simulink model "water_4hopper"  (Simulink 8.0)
settings: Solver=ode23  StartTime=0.0  StopTime=30  RelTol=1e-3
values from neighbouring files (symbols this model uses):
  Ac = [sum(Ay), sum(Ath), sum(Aph) ... (first row only)    [simpleSys.m]
  alpha = 1/16    (= 0.0625)    [simpleSys.m]
  C_d = 0.703    [simpleSys.m]
  density = 1000    [simpleSys.m]
  Filter_Coef = 1000    [simpleSys.m]
  g = 9.81    [simpleSys.m]
  Gc = [sum(G) - mass*g ; Lx'*G ; Lz'*G]    [simpleSys.m]
  mass = 0.15    [simpleSys.m]
  nullProj = eye(8) - pinvBc*Bc    [simpleSys.m]
  phi = 0 * pi/180    (= 0)    [simpleSys.m]
  pinvBc = pinv(Bc)    [simpleSys.m]
  S1 = pi*r1^2*area    (= 0.000684741534776)    [simpleSys.m]
  S2 = pi*r2^2*area    (= 4.27963459235e-05)    [simpleSys.m]
  theta = 0 * pi/180    (= 0)    [simpleSys.m]
  w = 60    [simpleSys.m]
  y = 0.020    (= 0.02)    [simpleSys.m]
undefined symbols (not defined in the file or in its folder): dTorqueAmp, dTorqueFreq, dTorquePhase, frame_inertia, freq, Kdf, leg_length, Mc, omega_0, tau, waveAmp, waveFreq
undefined symbols (not defined in the file): amp, cw_FL_HL, cw_FR_FL, cw_FR_HR, cw_HR_HL, FL_HL_lag, FR_FL_lag, FR_HR_lag, HR_HL_lag, K_d, K_i, K_p, wavePhase
libraries: mblibv1 x31, dspstat3 x6
(part 1 of 2)
settings Model: Creator=Metti  LastModifiedBy=nitisht  SimulationMode=accelerator
settings SolverCC: ZeroCrossControl=DisableAll
settings DataIOCC: SignalLoggingSaveFormat=ModelDataLogs
settings DebuggingCC: FcnCallInpInsideContextMsg=EnableAllAsWarning
settings SimMechanicsCC: VisSampleTime=0.05  AutoFitVis=GROWTOFIT  LastVizWinPosition=[1 41 1600 759]  CamPosition=[-6.20117;3.01965;9.86212;]  CamTarget=[-0.265896;0.0450483;0.16365;]  CamUpVector=[0.0887544;0.966202;-0.242026;]  CamHeight=0.984746  VisBackgroundColor=[0.9;0.9;0.95;]  DefaultBodyColor=[1;0;0;]
settings ConfigurationSet: Description=SimMechanics 2G

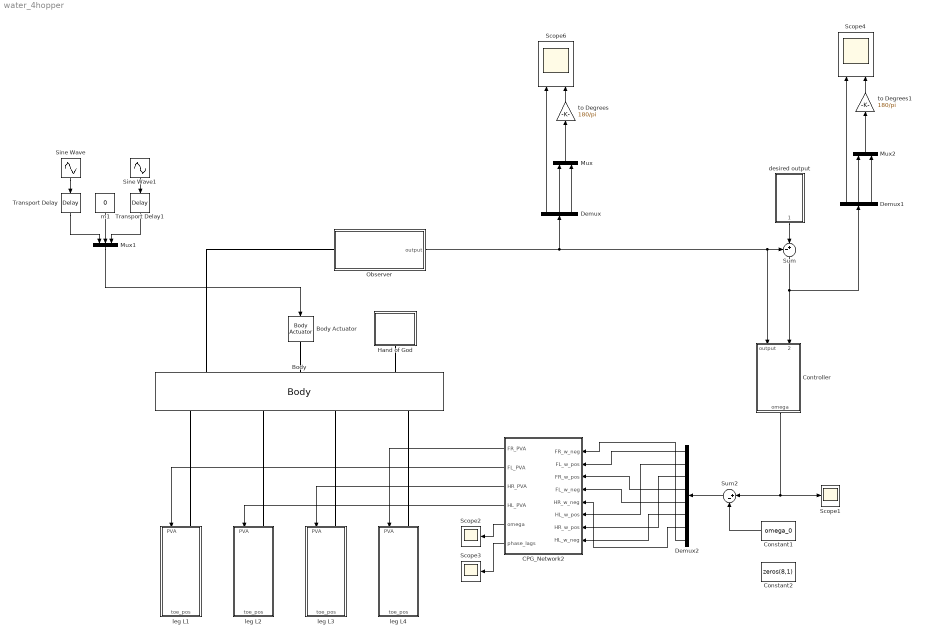
== system water_4hopper ==
  Body : mblibv1/Bodies/Body  LConnTagsString=CG|CS10|CS1  RConnTagsString=CS2|CS3|CS4|CS5  UpdateFromCAD=off  DialogClass=MechanicalBodyBlock  Mass=mass  MassUnits=kg  InertiaUnits=kg*m^2  Inertia=frame_inertia  Shape=Cylinder  ShapeDims=[1 1]  ShapeUnits=m  ShapeUse=false  Density=1  DensityUnits=kg/m^3  DensityUse=false  GraphicsMode=MACHINE_DEFAULT  BodyColorSelMode=MACHINE_DEFAULT  BodyColor=[1 0 0]  AttachedToCS=CG  CG=Left$CG$CG_pos$CS1$CS1$m$[0 0 0]$Euler X-Y-Z$deg$WORLD$true$none  WorkingFrames=Left$CS10$CG_pos$CS1$CS1$m$[0 0 0]$Euler X-Y-Z$deg$WORLD$true$none#Left$CS1$[0 0 0]$Adjoining$Adjoining$m$[0 0 0]$Euler X-Y-Z$deg$WORLD$true$none#Right$CS2$TR_FL$CS1$CS1$m$[0 0 0]$Euler X-Y-Z$deg$WORLD$true$none#Right$CS3$TR_HL$CS1$CS1$m$[0 0 0]$Euler X-Y-Z$deg$WORLD$true$none#Right$CS4$TR_HR$CS1$CS1$m$[0 0 0]$Euler X-Y-Z$deg$WORLD$true$none#Right$CS5$TR_FR$CS1$CS1$m$[0 0 0]$Euler X-Y-Z$deg$WORLD$true$none  CGPos=CG_pos  CGRot=[0 0 0]  CS0Pos=[]  CS0Rot=[]  CS1Pos=[0 0 0]  CS1Rot=[0 0 0]  CS2Pos=TR_FL  CS2Rot=[0 0 0]  CS3Pos=TR_HL  CS3Rot=[0 0 0]  CS4Pos=TR_HR  CS4Rot=[0 0 0]  CS5Pos=TR_FR  CS5Rot=[0 0 0]  CS6Pos=[]  CS6Rot=[]  CS7Pos=[]  CS7Rot=[]  CS8Pos=[]  CS8Rot=[]  CS9Pos=[]  CS9Rot=[]  CS10Pos=CG_pos  CS10Rot=[0 0 0]  CS11Pos=[]  CS11Rot=[]  CS12Pos=[]  CS12Rot=[]  CS13Pos=[]  CS13Rot=[]  CS14Pos=[]  CS14Rot=[]  CS15Pos=[]  CS15Rot=[]  CS16Pos=[]  CS16Rot=[]  CS17Pos=[]  CS17Rot=[]  CS18Pos=[]  CS18Rot=[]  CS19Pos=[]  CS19Rot=[]  CS20Pos=[]  CS20Rot=[]
  Body Actuator : mblibv1/Sensors &  Actuators/Body Actuator  UpdateFromCAD=off  PhysicalDomain=Mechanical  PortType=blob  ActuationStyle=Force  AngleUnits=deg  ArcVelocityUnits=deg/s  ArcAccelerationUnits=deg/s^2  CoordPositionUnits=m  VelocityUnits=m/s  AccelerationUnits=m/s^2  ForceUnits=N  TorqueUnits=N*m  ActiveIO=on  Width=3  DialogClass=MechanicalActuatorBlock  ReferenceFrame=Absolute (World)  Angle=off  CoordPosition=on  Force=off  Torque=on
  CPG_Network2 : Subsystem
  Constant1 : Constant  Value=omega_0
  Constant2 : Constant  Value=zeros(8,1)
  Controller : Subsystem
  Demux : Demux  Outputs=3
  Demux1 : Demux  Outputs=3
  Demux2 : Demux  Outputs=8
  Hand of God : Subsystem
  Mux : Mux  Inputs=2
  Mux1 : Mux  Inputs=3
  Mux2 : Mux  Inputs=2
  Observer : Subsystem
  Scope1 : Scope
      settings: TimeRange=30  YMin=25  YMax=95  SaveName=command_omega
  Scope2 : Scope
      settings: ShowLegends=on  TimeRange=30  YMin=-10  YMax=120  SaveName=CPG_omega
  Scope3 : Scope
      settings: ShowLegends=on  TimeRange=30  YMin=0  YMax=6.5  SaveName=CPG_phase_lags
  Scope4 : Scope  NumInputPorts=2
      settings: TimeRange=30  YMin=0.0125~-0.0225  YMax=0.0275~0.02  SaveName=ball_position1
  Scope6 : Scope  NumInputPorts=2
      settings: TimeRange=30  YMin=0.0125~-0.0225  YMax=0.0275~0.02  SaveName=ball_position
  Sine Wave : Sin  Amplitude=dTorqueAmp  Frequency=dTorqueFreq  Phase=dTorquePhase(1)  SampleTime=0
  Sine Wave1 : Sin  Amplitude=dTorqueAmp  Frequency=dTorqueFreq  Phase=dTorquePhase(2)  SampleTime=0
  Sum : Sum  Inputs=-+|
  Sum2 : Sum  Inputs=|+-
  Transport Delay : TransportDelay  DelayTime=5
  Transport Delay1 : TransportDelay  DelayTime=5
  desired output : Subsystem
  leg L1 : Subsystem  mask{wphase=wavePhase(1)}
      mask prompts: wphase "wave phase"
  leg L2 : Subsystem  mask{wphase=wavePhase(2)}
      mask prompts: wphase "wave phase"
  leg L3 : Subsystem  mask{wphase=wavePhase(3)}
      mask prompts: wphase "wave phase"
  leg L4 : Subsystem  mask{wphase=wavePhase(4)}
      mask prompts: wphase "wave phase"
  m1 : Constant  Value=0
  to Degrees : Gain  Gain=180/pi
  to Degrees1 : Gain  Gain=180/pi
  wires:
  Demux2/1 -> CPG_Network2/2(FL_w_pos)
  Demux2/5 -> CPG_Network2/4(FL_w_neg)
  Demux2/2 -> CPG_Network2/6(HL_w_pos)
  Demux2/6 -> CPG_Network2/8(HL_w_neg)
  Demux2/3 -> CPG_Network2/7(HR_w_pos)
  Demux2/7 -> CPG_Network2/5(HR_w_neg)
  Demux2/4 -> CPG_Network2/3(FR_w_pos)
  Demux2/8 -> CPG_Network2/1(FR_w_neg)
  CPG_Network2/5(omega) -> Scope2/1
  Sine Wave/1 -> Transport Delay/1
  Mux1/1 -> Body Actuator/1
  Transport Delay/1 -> Mux1/1
  Transport Delay1/1 -> Mux1/3
  m1/1 -> Mux1/2
  Sine Wave1/1 -> Transport Delay1/1
  CPG_Network2/6("phase_lags ") -> Scope3/1
  desired output/1(desired output) -> Sum/2
  Controller/1(omega) -> Scope1/1, Sum2/1
  CPG_Network2/2(FL_PVA) -> leg L1/1(PVA)
  CPG_Network2/4(HL_PVA) -> leg L2/1(PVA)
  CPG_Network2/3(HR_PVA) -> leg L3/1(PVA)
  CPG_Network2/1(FR_PVA) -> leg L4/1(PVA)
  Constant1/1 -> Sum2/2
  Observer/1(output) -> Sum/1, Controller/1(output), Demux/1
  Demux/2 -> Mux/1
  Demux/3 -> Mux/2
  Mux/1 -> to Degrees/1
  to Degrees/1 -> Scope6/2
  Demux/1 -> Scope6/1
  Sum2/1 -> Demux2/1
  Sum/1 -> Demux1/1, Controller/2(output error)
  Demux1/2 -> Mux2/1
  Demux1/3 -> Mux2/2
  Mux2/1 -> to Degrees1/1
  to Degrees1/1 -> Scope4/2
  Demux1/1 -> Scope4/1
  connections:
  Hand of God/RConn1 -- Body/LConn3
  leg L4/LConn1 -- Body/RConn4
  leg L3/LConn1 -- Body/RConn3
  leg L2/LConn1 -- Body/RConn2
  leg L1/LConn1 -- Body/RConn1
  Body Actuator/RConn1 -- Body/LConn2
  Observer/LConn1 -- Body/LConn1

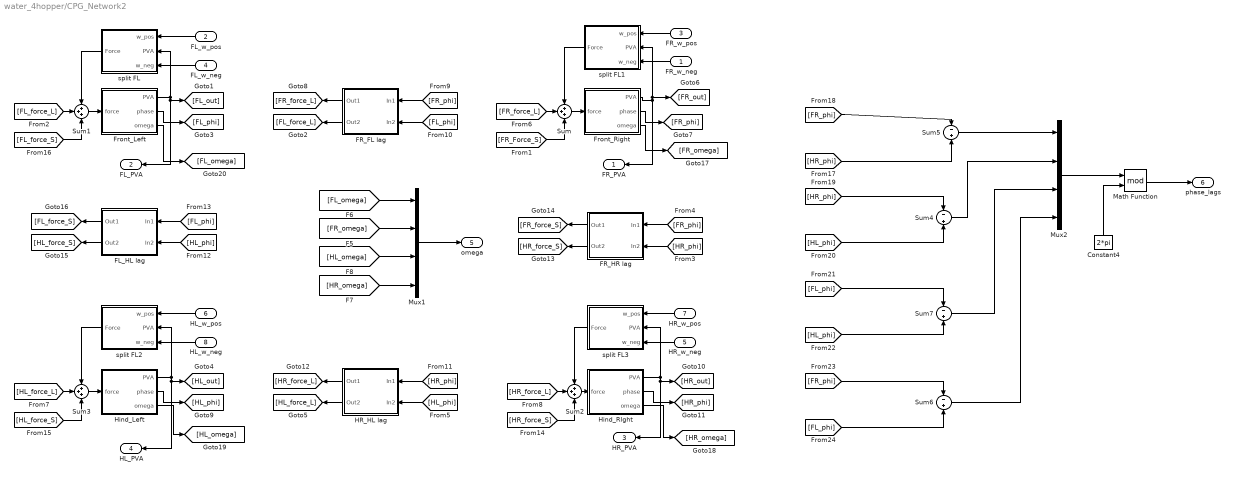
== system water_4hopper/CPG_Network2 ==
  FR_w_neg : Inport
  FL_w_pos : Inport  Port=2
  FR_w_pos : Inport  Port=3
  FL_w_neg : Inport  Port=4
  HR_w_neg : Inport  Port=5
  HL_w_pos : Inport  Port=6
  HR_w_pos : Inport  Port=7
  HL_w_neg : Inport  Port=8
  Constant4 : Constant  Value=2*pi
  FL_HL lag : Subsystem  mask{d_phase=FL_HL_lag, coupling_weight=cw_FL_HL}
      mask prompts: d_phase "Phase Lag"; coupling_weight "Coupling Weight"
  FR_FL lag : Subsystem  mask{d_phase=FR_FL_lag, coupling_weight=cw_FR_FL}
      mask prompts: d_phase "Phase Lag"; coupling_weight "Coupling Weight"
  FR_HR lag : Subsystem  mask{d_phase=FR_HR_lag, coupling_weight=cw_FR_HR}
      mask prompts: d_phase "Phase Lag"; coupling_weight "Coupling Weight"
  Front_Left : Subsystem  mask{Amp=amp, Offset=0, init_phi=pi}
      mask prompts: Amp "Amplitude"; init_phi "Initial Phase"
  Front_Right : Subsystem  mask{Amp=amp, Offset=0, init_phi=0}
      mask prompts: Amp "Amplitude"; init_phi "Initial Phase"
  HR_HL lag : Subsystem  mask{d_phase=HR_HL_lag, coupling_weight=cw_HR_HL}
      mask prompts: d_phase "Phase Lag"; coupling_weight "Coupling Weight"
  Hind_Left : Subsystem  mask{Amp=amp, Offset=0, init_phi=0}
      mask prompts: Amp "Amplitude"; init_phi "Initial Phase"
  Hind_RIght : Subsystem  mask{Amp=amp, Offset=0, init_phi=pi}
      mask prompts: Amp "Amplitude"; init_phi "Initial Phase"
  Math Function : Math  Operator=mod  SaturateOnIntegerOverflow=on
  Mux1 : Mux
  Mux2 : Mux
  Sum{,1..3} (4 alike) : Sum  Inputs=+++
  Sum{4..7} (4 alike) : Sum  Inputs=-|+
  split FL : Subsystem
  split FL1 : Subsystem
  split FL2 : Subsystem
  split FL3 : Subsystem
  FR_PVA : Outport
  FL_PVA : Outport  Port=2
  HR_PVA : Outport  Port=3
  HL_PVA : Outport  Port=4
  omega : Outport  Port=5
  "phase_lags " : Outport  Port=6
  wires:
  Front_Left/2(phase) -> [FL_phi]
  Front_Right/2(phase) -> [FR_phi]
  [FL_phi] -> FR_FL lag/2(In2)
  [FR_phi] -> FR_FL lag/1(In1)
  FR_FL lag/1(Out1) -> [FR_force_L]
  FR_FL lag/2(Out2) -> [FL_force_L]
  Front_Right/1(PVA) -> split FL1/2(PVA), [FR_out], FR_PVA/1
  [FL_force_L] -> Sum1/2
  Sum1/1 -> Front_Left/1(force)
  Sum/1 -> Front_Right/1(force)
  [FR_force_L] -> Sum/2
  FR_w_pos/1 -> split FL1/1(w_pos)
  FR_w_neg/1 -> split FL1/3(w_neg)
  split FL1/1(Force) -> Sum/1
  FL_w_pos/1 -> split FL/1(w_pos)
  FL_w_neg/1 -> split FL/3(w_neg)
  Front_Left/1(PVA) -> FL_PVA/1, [FL_out], split FL/2(PVA)
  split FL/1(Force) -> Sum1/1
  Hind_Left/2(phase) -> [HL_phi]
  Hind_RIght/2(phase) -> [HR_phi]
  [HL_phi] -> HR_HL lag/2(In2)
  [HR_phi] -> HR_HL lag/1(In1)
  HR_HL lag/1(Out1) -> [HR_force_L]
  HR_HL lag/2(Out2) -> [HL_force_L]
  Hind_RIght/1(PVA) -> HR_PVA/1, [HR_out], split FL3/2(PVA)
  [HL_force_L] -> Sum3/2
  Sum3/1 -> Hind_Left/1(force)
  Sum2/1 -> Hind_RIght/1(force)
  [HR_force_L] -> Sum2/2
  HR_w_pos/1 -> split FL3/1(w_pos)
  HR_w_neg/1 -> split FL3/3(w_neg)
  split FL3/1(Force) -> Sum2/1
  HL_w_pos/1 -> split FL2/1(w_pos)
  HL_w_neg/1 -> split FL2/3(w_neg)
  Hind_Left/1(PVA) -> HL_PVA/1, [HL_out], split FL2/2(PVA)
  split FL2/1(Force) -> Sum3/1
  [HR_phi] -> FR_HR lag/2(In2)
  [FR_phi] -> FR_HR lag/1(In1)
  FR_HR lag/1(Out1) -> [FR_force_S]
  FR_HR lag/2(Out2) -> [HR_force_S]
  [HL_phi] -> FL_HL lag/2(In2)
  [FL_phi] -> FL_HL lag/1(In1)
  FL_HL lag/1(Out1) -> [FL_force_S]
  FL_HL lag/2(Out2) -> [HL_force_S]
  [FR_Force_S] -> Sum/3
  [HR_force_S] -> Sum2/3
  [HL_force_S] -> Sum3/3
  [FL_force_S] -> Sum1/3
  Front_Right/3(omega) -> [FR_omega]
  Hind_RIght/3(omega) -> [HR_omega]
  Hind_Left/3(omega) -> [HL_omega]
  Front_Left/3(omega) -> [FL_omega]
  Mux1/1 -> omega/1
  [FR_omega] -> Mux1/2
  [FL_omega] -> Mux1/1
  [HL_omega] -> Mux1/3
  [HR_omega] -> Mux1/4
  Sum5/1 -> Mux2/1
  [HR_phi] -> Sum5/2
  [FR_phi] -> Sum5/1
  Sum4/1 -> Mux2/2
  [HR_phi] -> Sum4/1
  [HL_phi] -> Sum4/2
  [FL_phi] -> Sum7/1
  Sum6/1 -> Mux2/4
  [FR_phi] -> Sum6/1
  [FL_phi] -> Sum6/2
  Math Function/1 -> "phase_lags "/1
  Constant4/1 -> Math Function/2
  Mux2/1 -> Math Function/1
  Sum7/1 -> Mux2/3
  [HL_phi] -> Sum7/2

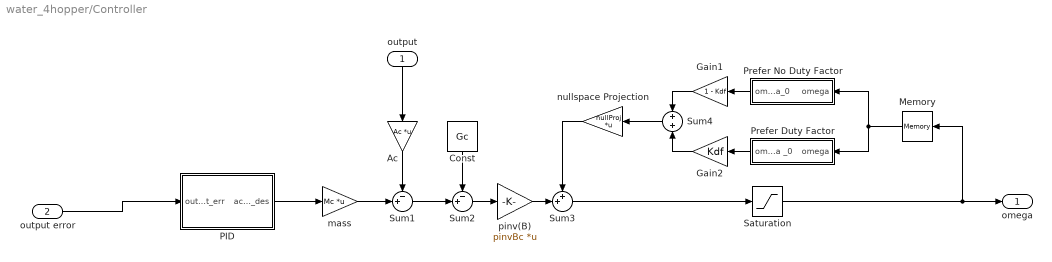
== system water_4hopper/Controller ==
  output : Inport
  output error : Inport  Port=2
  Ac : Gain  Gain=Ac  Multiplication=Matrix(K*u)
  Const : Constant  Value=Gc
  Gain1 : Gain  Gain=1 - Kdf
  Gain2 : Gain  Gain=Kdf
  Memory : Memory  X0=w*ones(8,1)
  PID : Subsystem  mask{P=K_p, I=K_i, D=K_d, N=Filter_Coef}
      mask prompts: P "Proportional Gain"; I "Integral Gain"; D "Derivative Gain"; N "Filter Coefficient"
  Prefer Duty Factor : Subsystem
  Prefer No Duty Factor : Subsystem
  Saturation : Saturate  UpperLimit=120  LowerLimit=10
  Sum1 : Sum  Inputs=-+|
  Sum2 : Sum  Inputs=-+|
  Sum3 : Sum  Inputs=++|
  Sum4 : Sum  Inputs=+|+
  mass : Gain  Gain=Mc  Multiplication=Matrix(K*u)
  nullspace Projection : Gain  Gain=nullProj  Multiplication=Matrix(K*u)
  pinv(B) : Gain  Gain=pinvBc  Multiplication=Matrix(K*u)
  omega : Outport
  wires:
  Gain2/1 -> Sum4/2
  output/1 -> Ac/1
  Sum2/1 -> pinv(B)/1
  mass/1 -> Sum1/2
  Memory/1 -> Prefer Duty Factor/1(omega), Prefer No Duty Factor/1(omega)
  Prefer No Duty Factor/1(omega_0) -> Gain1/1
  Prefer Duty Factor/1(omega _0) -> Gain2/1
  Gain1/1 -> Sum4/1
  output error/1 -> PID/1(output_err)
  Sum3/1 -> Saturation/1
  Sum4/1 -> nullspace Projection/1
  Saturation/1 -> Memory/1, omega/1
  Ac/1 -> Sum1/1
  pinv(B)/1 -> Sum3/2
  nullspace Projection/1 -> Sum3/1
  Sum1/1 -> Sum2/2
  Const/1 -> Sum2/1
  PID/1(accel_des) -> mass/1

== system water_4hopper/Hand of God ==
  Custom Joint : mblibv1/Joints/Custom Joint  LConnTagsString=__newl0|SA1  RConnTagsString=__newr0  UpdateFromCAD=off  NumSAPorts=1  CutJoint=off  MarkAsCut=off  Primitives=prismatic  PrimitiveProps=P1$World$[0 1 0]$Prismatic#R1$World$[1 0 0]$Revolute#R2$World$[0 0 1]$Revolute  DialogClass=JointBlock  R1Axis=[1 0 0]  R2Axis=[0 0 1]  R3Axis=[]  P1Axis=[0 1 0]  P2Axis=[]  P3Axis=[]  SAxis=[]
  Ground : mblibv1/Bodies/Ground  UpdateFromCAD=off  LeftPortType=env  RightPortType=workingframe  PhysicalDomain=Mechanical  DialogClass=GroundBlock  CoordPosition=[0 0 0]  CoordPositionUnits=m  StateVectorMgrId=0  MachineId=[1 0]  ShowEnvPort=on
  Joint Initial Condition : mblibv1/Sensors &  Actuators/Joint Initial Condition  UpdateFromCAD=off  LeftPortType=blob  RightPortType=blob  PhysicalDomain=mechanical  DialogClass=InitialConditionBlock  InitialConditions=P1$true$y$m$deg$0$m/s$deg/s#P2$false$0$m$deg$0$m/s$deg/s#P3$false$0$m$deg$0$m/s$deg/s#R1$true$0$m$deg$0$m/s$deg/s#R2$true$0$m$deg$0$m/s$deg/s#R3$false$10$m$deg$0$m/s$deg/s#S$false$0$m$deg$0$m/s$deg/s  P1PIC=y  P1VIC=0  P2PIC=0  P2VIC=0  P3PIC=0  P3VIC=0  R1PIC=0  R1VIC=0  R2PIC=0  R2VIC=0  R3PIC=0  R3VIC=0  SPIC=0  SVIC=0
  Joint Sensor : mblibv1/Sensors &  Actuators/Joint Sensor  UpdateFromCAD=off  PhysicalDomain=Mechanical  PortType=blob  Muxed=on  Pose=off  Angle=on  AngleUnits=deg  ArcVelocity=off  ArcVelocityUnits=deg/s  ArcAcceleration=off  ArcAccelerationUnits=deg/s^2  CoordPosition=on  CoordPositionUnits=m  Velocity=off  VelocityUnits=m/s  Acceleration=off  AccelerationUnits=m/s^2  Quaternion=on  QuaternionDT=off  QuaternionDDT=off  QuaternionUnits=off  OutputVector=[1]  ActiveIO=on  Width=1  DialogClass=MechanicalSensorBlock  Primitive=P1  Force=off  ForceUnits=N  Torque=off  TorqueUnits=N*m  ReferenceFrame=Absolute (World)  ReactionSensedSide=Base  ReactionReferenceFrame=Absolute (World)  ReactionForce=off  ReactionForceUnits=N  ReactionMoment=off  ReactionMomentUnits=N*m
  Joint Sensor1 : mblibv1/Sensors &  Actuators/Joint Sensor  UpdateFromCAD=off  PhysicalDomain=Mechanical  PortType=blob  Muxed=on  Pose=off  Angle=on  AngleUnits=deg  ArcVelocity=off  ArcVelocityUnits=deg/s  ArcAcceleration=off  ArcAccelerationUnits=deg/s^2  CoordPosition=off  CoordPositionUnits=m  Velocity=on  VelocityUnits=m/s  Acceleration=off  AccelerationUnits=m/s^2  Quaternion=on  QuaternionDT=off  QuaternionDDT=off  QuaternionUnits=off  OutputVector=[1]  ActiveIO=on  Width=1  DialogClass=MechanicalSensorBlock  Primitive=R1  Force=off  ForceUnits=N  Torque=off  TorqueUnits=N*m  ReferenceFrame=Absolute (World)  ReactionSensedSide=Base  ReactionReferenceFrame=Absolute (World)  ReactionForce=off  ReactionForceUnits=N  ReactionMoment=off  ReactionMomentUnits=N*m
  Joint Sensor2 : mblibv1/Sensors &  Actuators/Joint Sensor  UpdateFromCAD=off  PhysicalDomain=Mechanical  PortType=blob  Muxed=off  Pose=off  Angle=on  AngleUnits=deg  ArcVelocity=off  ArcVelocityUnits=deg/s  ArcAcceleration=off  ArcAccelerationUnits=deg/s^2  CoordPosition=on  CoordPositionUnits=m  Velocity=off  VelocityUnits=m/s  Acceleration=off  AccelerationUnits=m/s^2  Quaternion=on  QuaternionDT=off  QuaternionDDT=off  QuaternionUnits=off  OutputVector=[1]  ActiveIO=on  Width=1  DialogClass=MechanicalSensorBlock  Primitive=R2  Force=off  ForceUnits=N  Torque=off  TorqueUnits=N*m  ReferenceFrame=Absolute (World)  ReactionSensedSide=Base  ReactionReferenceFrame=Absolute (World)  ReactionForce=off  ReactionForceUnits=N  ReactionMoment=off  ReactionMomentUnits=N*m
  Machine Environment : mblibv1/Bodies/Machine Environment  PortType=env  PhysicalDomain=Mechanical  DialogTemplateClass=MECH.MachineEnvironment  SyncWhenCopied=off  Gravity=[0 -g 0]  GravityUnits=m/s^2  GravityAsSignal=off  Dimensionality=Auto-detect  AnalysisType=Forward dynamics  LinearAssemblyTolerance=1e-3  LinearAssemblyToleranceUnits=m  AngularAssemblyTolerance=1e-3  AngularAssemblyToleranceUnits=rad  ConstraintSolverType=Stabilizing  ConstraintRelTolerance=1e-4  ConstraintAbsTolerance=1e-4  UseRobustSingularityHandling=off  RedundancyAnalysisToleranceType=Automatically select tolerance  RedundancyAnalysisTolerance=1e-14  StatePerturbationType=Fixed  PerturbationSize=1e-5  VisualizeMachine=on  BodyVisualizationType=Use model default body geometries  BodyColorSelMode=Use model default  DefaultBodyColor=[1 0 0]
  Mechanical Branching Bar : mblibv1/Utilities/Mechanical Branching Bar  LConnTagsString=_newl0  RConnTagsString=__newr0|SA2|SA3|SA4  UpdateFromCAD=off  DialogClass=MechanicalBranchingBarBlock  NumSAPorts=4
  Scope : Scope  NumInputPorts=3
      settings: TimeRange=5  YMin=-0.01~-0.001~-6  YMax=0.02~0.0004~1  SaveName=mass_data
  Conn1 : PMIOPort  Port=1  Side=Right
  wires:
  Joint Sensor/1 -> Scope/1
  Joint Sensor1/1 -> Scope/2
  Joint Sensor2/1 -> Scope/3
  connections:
  Conn1/RConn1 -- Custom Joint/RConn1
  Joint Sensor1/LConn1 -- Mechanical Branching Bar/RConn3
  Ground/RConn1 -- Custom Joint/LConn1
  Machine Environment/RConn1 -- Ground/LConn1
  Joint Initial Condition/RConn1 -- Mechanical Branching Bar/RConn1
  Joint Sensor/LConn1 -- Mechanical Branching Bar/RConn2
  Custom Joint/LConn2 -- Mechanical Branching Bar/LConn1
  Joint Sensor2/LConn1 -- Mechanical Branching Bar/RConn4

== system water_4hopper/Observer ==
  Body Sensor5 : mblibv1/Sensors &  Actuators/Body Sensor  UpdateFromCAD=off  PhysicalDomain=Mechanical  PortType=blob  Muxed=off  Pose=off  Angle=on  AngleUnits=deg  ArcVelocity=on  ArcVelocityUnits=rad/s  ArcAcceleration=off  ArcAccelerationUnits=rad/s^2  CoordPosition=on  CoordPositionUnits=m  Velocity=off  VelocityUnits=m/s  Acceleration=off  AccelerationUnits=m/s^2  Quaternion=on  QuaternionDT=off  QuaternionDDT=off  QuaternionUnits=off  OutputVector=[1]  ActiveIO=on  Width=6  DialogClass=MechanicalSensorBlock  ReferenceFrame=Absolute (World)
  Gain1 : Gain  Gain=-1
  Integrator1 : Integrator
  Mux : Mux  Inputs=2
  Selector5 : Selector  InputPortWidth=3  IndexOptions=Index vector (dialog)  Indices=[2]  OutputSizes=1
  Selector6 : Selector  InputPortWidth=3  IndexOptions=Index vector (dialog)  Indices=[1 3]  OutputSizes=1
  averaging2 : Subsystem  mask{T_win=2*pi/freq*4, x_init=y}
      mask prompts: T_win "window (s)"; x_init "Initial condition"
  averaging4 : Subsystem  mask{T_win=2*pi/freq*4, x_init=[0 0]}
      mask prompts: T_win "window (s)"; x_init "Initial condition"
  Body : PMIOPort  Port=1  Side=Left
  output : Outport
  wires:
  Gain1/1 -> Mux/2
  Body Sensor5/1 -> Selector5/1
  Selector6/1 -> averaging4/1(in)
  Body Sensor5/2 -> Integrator1/1
  averaging2/1(out) -> Mux/1
  Mux/1 -> output/1
  averaging4/1(out) -> Gain1/1
  Selector5/1 -> averaging2/1(in)
  Integrator1/1 -> Selector6/1
  connections:
  Body Sensor5/LConn1 -- Body/RConn1

== system water_4hopper/desired output ==
  Mux : Mux  Inputs=2
  Mux1 : Mux  Inputs=2
  Step : Step  Time=5  After=theta  SampleTime=0
  Step1 : Step  Time=10  After=-2*theta  SampleTime=0
  Step2 : Step  Time=15  After=theta  SampleTime=0
  Step3 : Step  Time=5  After=phi  SampleTime=0
  Step4 : Step  Time=10  After=-2*phi  SampleTime=0
  Step5 : Step  Time=15  After=phi  SampleTime=0
  Sum1 : Sum  Inputs=+++
  Sum3 : Sum  Inputs=+++
  m : Constant  Value=y
  desired output : Outport
  wires:
  m/1 -> Mux1/1  "height"
  Step/1 -> Sum1/1
  Step1/1 -> Sum1/2
  Step2/1 -> Sum1/3
  Step4/1 -> Sum3/2
  Step3/1 -> Sum3/1
  Step5/1 -> Sum3/3
  Sum1/1 -> Mux/1  "roll"
  Sum3/1 -> Mux/2  "pitch"
  Mux/1 -> Mux1/2
  Mux1/1 -> desired output/1

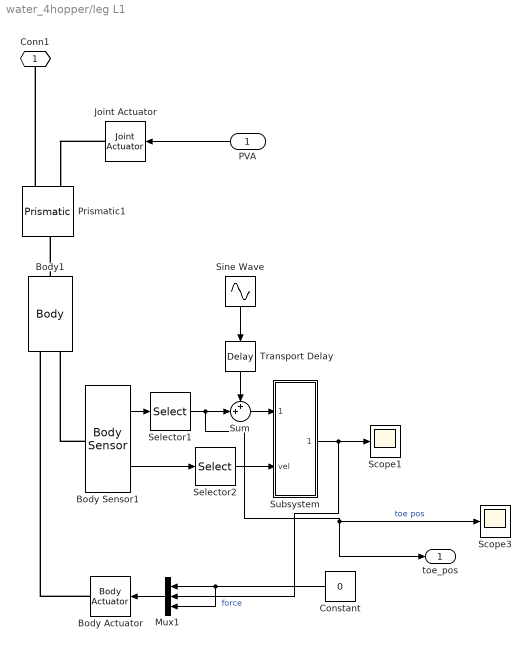
== system water_4hopper/leg L1 ==
  PVA : Inport
  Body Actuator : mblibv1/Sensors &  Actuators/Body Actuator  UpdateFromCAD=off  PhysicalDomain=Mechanical  PortType=blob  ActuationStyle=Force  AngleUnits=deg  ArcVelocityUnits=deg/s  ArcAccelerationUnits=deg/s^2  CoordPositionUnits=m  VelocityUnits=m/s  AccelerationUnits=m/s^2  ForceUnits=N  TorqueUnits=N*m  ActiveIO=on  Width=3  DialogClass=MechanicalActuatorBlock  ReferenceFrame=Local (Body CS)  Angle=off  CoordPosition=on  Force=on  Torque=off
  Body Sensor1 : mblibv1/Sensors &  Actuators/Body Sensor  UpdateFromCAD=off  PhysicalDomain=Mechanical  PortType=blob  Muxed=off  Pose=off  Angle=on  AngleUnits=deg  ArcVelocity=off  ArcVelocityUnits=deg/s  ArcAcceleration=off  ArcAccelerationUnits=deg/s^2  CoordPosition=on  CoordPositionUnits=m  Velocity=on  VelocityUnits=m/s  Acceleration=off  AccelerationUnits=m/s^2  Quaternion=on  QuaternionDT=off  QuaternionDDT=off  QuaternionUnits=off  OutputVector=[1]  ActiveIO=on  Width=6  DialogClass=MechanicalSensorBlock  ReferenceFrame=Absolute (World)
  Body1 : mblibv1/Bodies/Body  LConnTagsString=CS1  RConnTagsString=CS2|CS3  UpdateFromCAD=off  DialogClass=MechanicalBodyBlock  Mass=0  MassUnits=kg  InertiaUnits=kg*m^2  Inertia=zeros(3)  Shape=Cylinder  ShapeDims=[1 1]  ShapeUnits=m  ShapeUse=false  Density=1  DensityUnits=kg/m^3  DensityUse=false  GraphicsMode=MACHINE_DEFAULT  BodyColorSelMode=MACHINE_DEFAULT  BodyColor=[1 0 0]  AttachedToCS=CG  CG=Left$CG$[0 -leg_length 0]$CS1$CS1$m$[0 0 0]$Euler X-Y-Z$deg$WORLD$false$none  WorkingFrames=Left$CS1$[0 0 0]$Adjoining$Adjoining$m$[0 0 0]$Euler X-Y-Z$deg$WORLD$true$none#Right$CS2$[0 -leg_length 0]$CS1$CS1$m$[0 0 0]$Euler X-Y-Z$deg$WORLD$true$none#Right$CS3$[0 -leg_length 0]$CS1$CS1$m$[0 0 0]$Euler X-Y-Z$deg$WORLD$true$none  CGPos=[0 -leg_length 0]  CGRot=[0 0 0]  CS0Pos=[]  CS0Rot=[]  CS1Pos=[0 0 0]  CS1Rot=[0 0 0]  CS2Pos=[0 -leg_length 0]  CS2Rot=[0 0 0]  CS3Pos=[0 -leg_length 0]  CS3Rot=[0 0 0]  CS4Pos=[]  CS4Rot=[]  CS5Pos=[]  CS5Rot=[]  CS6Pos=[]  CS6Rot=[]  CS7Pos=[]  CS7Rot=[]  CS8Pos=[]  CS8Rot=[]  CS9Pos=[]  CS9Rot=[]  CS10Pos=[]  CS10Rot=[]  CS11Pos=[]  CS11Rot=[]  CS12Pos=[]  CS12Rot=[]  CS13Pos=[]  CS13Rot=[]  CS14Pos=[]  CS14Rot=[]  CS15Pos=[]  CS15Rot=[]  CS16Pos=[]  CS16Rot=[]  CS17Pos=[]  CS17Rot=[]  CS18Pos=[]  CS18Rot=[]  CS19Pos=[]  CS19Rot=[]  CS20Pos=[]  CS20Rot=[]
  Constant : Constant  Value=0
  Joint Actuator : mblibv1/Sensors &  Actuators/Joint Actuator  UpdateFromCAD=off  PhysicalDomain=Mechanical  PortType=blob  ActuationStyle=Motion  AngleUnits=deg  ArcVelocityUnits=deg/s  ArcAccelerationUnits=deg/s^2  CoordPositionUnits=m  VelocityUnits=m/s  AccelerationUnits=m/s^2  ForceUnits=N  TorqueUnits=N*m  ActiveIO=on  Width=3  DialogClass=MechanicalActuatorBlock  Primitive=P1  ReferenceFrame=Absolute (World)
  Mux1 : Mux  Inputs=3
  Prismatic1 : mblibv1/Joints/Prismatic  LConnTagsString=__newl0|SA1  RConnTagsString=__newr0  UpdateFromCAD=off  NumSAPorts=1  CutJoint=off  MarkAsCut=off  Primitives=prismatic  PrimitiveProps=P1$World$[0 1 0]$prismatic  DialogClass=JointBlock  P1Axis=[0 1 0]
  Scope1 : Scope
      settings: SaveName=force_L
  Scope3 : Scope
      settings: SaveName=toe_position_L
  Selector1 : Selector  InputPortWidth=3  IndexOptions=Index vector (dialog)  Indices=[2]  OutputSizes=1
  Selector2 : Selector  InputPortWidth=3  IndexOptions=Index vector (dialog)  Indices=[2]  OutputSizes=1
  Sine Wave : Sin  Amplitude=waveAmp  Frequency=waveFreq  Phase=wphase  SampleTime=0
  Subsystem : Subsystem
  Sum : Sum  Inputs=++|
  Transport Delay : TransportDelay  DelayTime=5
  Conn1 : PMIOPort  Port=1  Side=Left
  toe_pos : Outport
  wires:
  Body Sensor1/2 -> Selector2/1
  Selector1/1 -> Sum/2, Scope3/1, toe_pos/1  "toe pos"
  Selector2/1 -> Subsystem/2(vel)
  Subsystem/1(force) -> Scope1/1, Mux1/2  "force"
  Mux1/1 -> Body Actuator/1
  Constant/1 -> Mux1/1, Mux1/3
  PVA/1 -> Joint Actuator/1
  Body Sensor1/1 -> Selector1/1
  Sine Wave/1 -> Transport Delay/1
  Sum/1 -> Subsystem/1(pos)
  Transport Delay/1 -> Sum/1
  connections:
  Body1/LConn1 -- Prismatic1/RConn1
  Body Actuator/RConn1 -- Body1/RConn1
  Body Sensor1/LConn1 -- Body1/RConn2
  Prismatic1/LConn1 -- Conn1/RConn1
  Joint Actuator/RConn1 -- Prismatic1/LConn2

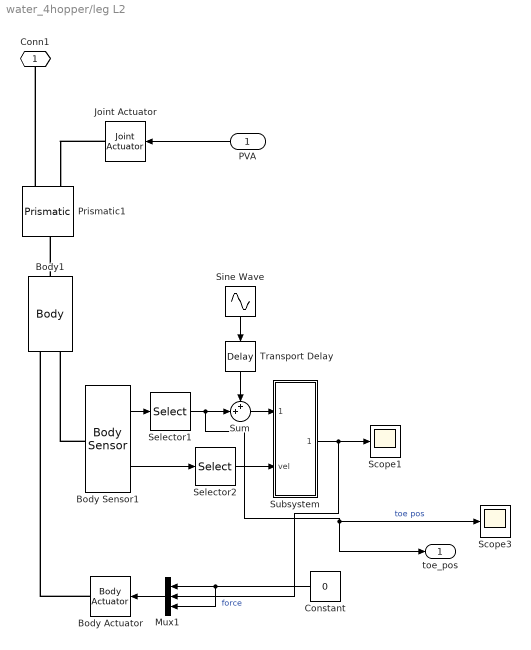
== system water_4hopper/leg L2 ==
  PVA : Inport
  Body Actuator : mblibv1/Sensors &  Actuators/Body Actuator  UpdateFromCAD=off  PhysicalDomain=Mechanical  PortType=blob  ActuationStyle=Force  AngleUnits=deg  ArcVelocityUnits=deg/s  ArcAccelerationUnits=deg/s^2  CoordPositionUnits=m  VelocityUnits=m/s  AccelerationUnits=m/s^2  ForceUnits=N  TorqueUnits=N*m  ActiveIO=on  Width=3  DialogClass=MechanicalActuatorBlock  ReferenceFrame=Local (Body CS)  Angle=off  CoordPosition=on  Force=on  Torque=off
  Body Sensor1 : mblibv1/Sensors &  Actuators/Body Sensor  UpdateFromCAD=off  PhysicalDomain=Mechanical  PortType=blob  Muxed=off  Pose=off  Angle=on  AngleUnits=deg  ArcVelocity=off  ArcVelocityUnits=deg/s  ArcAcceleration=off  ArcAccelerationUnits=deg/s^2  CoordPosition=on  CoordPositionUnits=m  Velocity=on  VelocityUnits=m/s  Acceleration=off  AccelerationUnits=m/s^2  Quaternion=on  QuaternionDT=off  QuaternionDDT=off  QuaternionUnits=off  OutputVector=[1]  ActiveIO=on  Width=6  DialogClass=MechanicalSensorBlock  ReferenceFrame=Absolute (World)
  Body1 : mblibv1/Bodies/Body  LConnTagsString=CS1  RConnTagsString=CS2|CS3  UpdateFromCAD=off  DialogClass=MechanicalBodyBlock  Mass=0  MassUnits=kg  InertiaUnits=kg*m^2  Inertia=zeros(3)  Shape=Cylinder  ShapeDims=[1 1]  ShapeUnits=m  ShapeUse=false  Density=1  DensityUnits=kg/m^3  DensityUse=false  GraphicsMode=MACHINE_DEFAULT  BodyColorSelMode=MACHINE_DEFAULT  BodyColor=[1 0 0]  AttachedToCS=CG  CG=Left$CG$[0 -leg_length 0]$CS1$CS1$m$[0 0 0]$Euler X-Y-Z$deg$WORLD$false$none  WorkingFrames=Left$CS1$[0 0 0]$Adjoining$Adjoining$m$[0 0 0]$Euler X-Y-Z$deg$WORLD$true$none#Right$CS2$[0 -leg_length 0]$CS1$CS1$m$[0 0 0]$Euler X-Y-Z$deg$WORLD$true$none#Right$CS3$[0 -leg_length 0]$CS1$CS1$m$[0 0 0]$Euler X-Y-Z$deg$WORLD$true$none  CGPos=[0 -leg_length 0]  CGRot=[0 0 0]  CS0Pos=[]  CS0Rot=[]  CS1Pos=[0 0 0]  CS1Rot=[0 0 0]  CS2Pos=[0 -leg_length 0]  CS2Rot=[0 0 0]  CS3Pos=[0 -leg_length 0]  CS3Rot=[0 0 0]  CS4Pos=[]  CS4Rot=[]  CS5Pos=[]  CS5Rot=[]  CS6Pos=[]  CS6Rot=[]  CS7Pos=[]  CS7Rot=[]  CS8Pos=[]  CS8Rot=[]  CS9Pos=[]  CS9Rot=[]  CS10Pos=[]  CS10Rot=[]  CS11Pos=[]  CS11Rot=[]  CS12Pos=[]  CS12Rot=[]  CS13Pos=[]  CS13Rot=[]  CS14Pos=[]  CS14Rot=[]  CS15Pos=[]  CS15Rot=[]  CS16Pos=[]  CS16Rot=[]  CS17Pos=[]  CS17Rot=[]  CS18Pos=[]  CS18Rot=[]  CS19Pos=[]  CS19Rot=[]  CS20Pos=[]  CS20Rot=[]
  Constant : Constant  Value=0
  Joint Actuator : mblibv1/Sensors &  Actuators/Joint Actuator  UpdateFromCAD=off  PhysicalDomain=Mechanical  PortType=blob  ActuationStyle=Motion  AngleUnits=deg  ArcVelocityUnits=deg/s  ArcAccelerationUnits=deg/s^2  CoordPositionUnits=m  VelocityUnits=m/s  AccelerationUnits=m/s^2  ForceUnits=N  TorqueUnits=N*m  ActiveIO=on  Width=3  DialogClass=MechanicalActuatorBlock  Primitive=P1  ReferenceFrame=Absolute (World)
  Mux1 : Mux  Inputs=3
  Prismatic1 : mblibv1/Joints/Prismatic  LConnTagsString=__newl0|SA1  RConnTagsString=__newr0  UpdateFromCAD=off  NumSAPorts=1  CutJoint=off  MarkAsCut=off  Primitives=prismatic  PrimitiveProps=P1$World$[0 1 0]$prismatic  DialogClass=JointBlock  P1Axis=[0 1 0]
  Scope1 : Scope
      settings: SaveName=force_L
  Scope3 : Scope
      settings: SaveName=toe_position_L
  Selector1 : Selector  InputPortWidth=3  IndexOptions=Index vector (dialog)  Indices=[2]  OutputSizes=1
  Selector2 : Selector  InputPortWidth=3  IndexOptions=Index vector (dialog)  Indices=[2]  OutputSizes=1
  Sine Wave : Sin  Amplitude=waveAmp  Frequency=waveFreq  Phase=wphase  SampleTime=0
  Subsystem : Subsystem
  Sum : Sum  Inputs=++|
  Transport Delay : TransportDelay  DelayTime=5
  Conn1 : PMIOPort  Port=1  Side=Left
  toe_pos : Outport
  wires:
  Body Sensor1/2 -> Selector2/1
  Selector1/1 -> Sum/2, Scope3/1, toe_pos/1  "toe pos"
  Selector2/1 -> Subsystem/2(vel)
  Subsystem/1(force) -> Scope1/1, Mux1/2  "force"
  Mux1/1 -> Body Actuator/1
  Constant/1 -> Mux1/1, Mux1/3
  PVA/1 -> Joint Actuator/1
  Body Sensor1/1 -> Selector1/1
  Sine Wave/1 -> Transport Delay/1
  Sum/1 -> Subsystem/1(pos)
  Transport Delay/1 -> Sum/1
  connections:
  Body1/LConn1 -- Prismatic1/RConn1
  Body Actuator/RConn1 -- Body1/RConn1
  Body Sensor1/LConn1 -- Body1/RConn2
  Prismatic1/LConn1 -- Conn1/RConn1
  Joint Actuator/RConn1 -- Prismatic1/LConn2

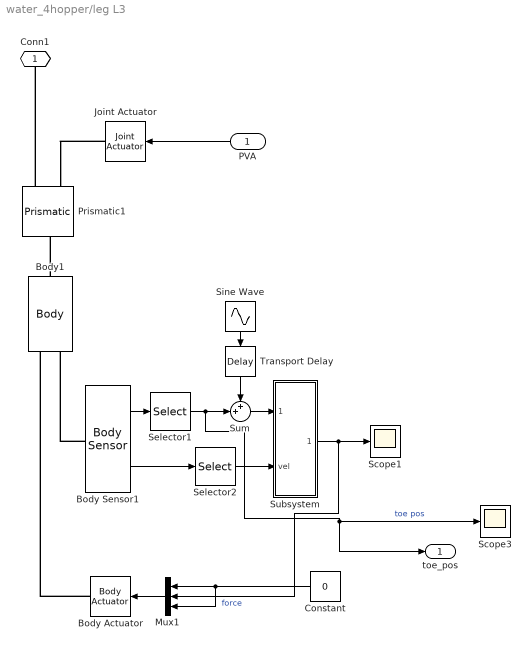
== system water_4hopper/leg L3 ==
  PVA : Inport
  Body Actuator : mblibv1/Sensors &  Actuators/Body Actuator  UpdateFromCAD=off  PhysicalDomain=Mechanical  PortType=blob  ActuationStyle=Force  AngleUnits=deg  ArcVelocityUnits=deg/s  ArcAccelerationUnits=deg/s^2  CoordPositionUnits=m  VelocityUnits=m/s  AccelerationUnits=m/s^2  ForceUnits=N  TorqueUnits=N*m  ActiveIO=on  Width=3  DialogClass=MechanicalActuatorBlock  ReferenceFrame=Local (Body CS)  Angle=off  CoordPosition=on  Force=on  Torque=off
  Body Sensor1 : mblibv1/Sensors &  Actuators/Body Sensor  UpdateFromCAD=off  PhysicalDomain=Mechanical  PortType=blob  Muxed=off  Pose=off  Angle=on  AngleUnits=deg  ArcVelocity=off  ArcVelocityUnits=deg/s  ArcAcceleration=off  ArcAccelerationUnits=deg/s^2  CoordPosition=on  CoordPositionUnits=m  Velocity=on  VelocityUnits=m/s  Acceleration=off  AccelerationUnits=m/s^2  Quaternion=on  QuaternionDT=off  QuaternionDDT=off  QuaternionUnits=off  OutputVector=[1]  ActiveIO=on  Width=6  DialogClass=MechanicalSensorBlock  ReferenceFrame=Absolute (World)
  Body1 : mblibv1/Bodies/Body  LConnTagsString=CS1  RConnTagsString=CS2|CS3  UpdateFromCAD=off  DialogClass=MechanicalBodyBlock  Mass=0  MassUnits=kg  InertiaUnits=kg*m^2  Inertia=zeros(3)  Shape=Cylinder  ShapeDims=[1 1]  ShapeUnits=m  ShapeUse=false  Density=1  DensityUnits=kg/m^3  DensityUse=false  GraphicsMode=MACHINE_DEFAULT  BodyColorSelMode=MACHINE_DEFAULT  BodyColor=[1 0 0]  AttachedToCS=CG  CG=Left$CG$[0 -leg_length 0]$CS1$CS1$m$[0 0 0]$Euler X-Y-Z$deg$WORLD$false$none  WorkingFrames=Left$CS1$[0 0 0]$Adjoining$Adjoining$m$[0 0 0]$Euler X-Y-Z$deg$WORLD$true$none#Right$CS2$[0 -leg_length 0]$CS1$CS1$m$[0 0 0]$Euler X-Y-Z$deg$WORLD$true$none#Right$CS3$[0 -leg_length 0]$CS1$CS1$m$[0 0 0]$Euler X-Y-Z$deg$WORLD$true$none  CGPos=[0 -leg_length 0]  CGRot=[0 0 0]  CS0Pos=[]  CS0Rot=[]  CS1Pos=[0 0 0]  CS1Rot=[0 0 0]  CS2Pos=[0 -leg_length 0]  CS2Rot=[0 0 0]  CS3Pos=[0 -leg_length 0]  CS3Rot=[0 0 0]  CS4Pos=[]  CS4Rot=[]  CS5Pos=[]  CS5Rot=[]  CS6Pos=[]  CS6Rot=[]  CS7Pos=[]  CS7Rot=[]  CS8Pos=[]  CS8Rot=[]  CS9Pos=[]  CS9Rot=[]  CS10Pos=[]  CS10Rot=[]  CS11Pos=[]  CS11Rot=[]  CS12Pos=[]  CS12Rot=[]  CS13Pos=[]  CS13Rot=[]  CS14Pos=[]  CS14Rot=[]  CS15Pos=[]  CS15Rot=[]  CS16Pos=[]  CS16Rot=[]  CS17Pos=[]  CS17Rot=[]  CS18Pos=[]  CS18Rot=[]  CS19Pos=[]  CS19Rot=[]  CS20Pos=[]  CS20Rot=[]
  Constant : Constant  Value=0
  Joint Actuator : mblibv1/Sensors &  Actuators/Joint Actuator  UpdateFromCAD=off  PhysicalDomain=Mechanical  PortType=blob  ActuationStyle=Motion  AngleUnits=deg  ArcVelocityUnits=deg/s  ArcAccelerationUnits=deg/s^2  CoordPositionUnits=m  VelocityUnits=m/s  AccelerationUnits=m/s^2  ForceUnits=N  TorqueUnits=N*m  ActiveIO=on  Width=3  DialogClass=MechanicalActuatorBlock  Primitive=P1  ReferenceFrame=Absolute (World)
  Mux1 : Mux  Inputs=3
  Prismatic1 : mblibv1/Joints/Prismatic  LConnTagsString=__newl0|SA1  RConnTagsString=__newr0  UpdateFromCAD=off  NumSAPorts=1  CutJoint=off  MarkAsCut=off  Primitives=prismatic  PrimitiveProps=P1$World$[0 1 0]$prismatic  DialogClass=JointBlock  P1Axis=[0 1 0]
  Scope1 : Scope
      settings: SaveName=force_L
  Scope3 : Scope
      settings: SaveName=toe_position_L
  Selector1 : Selector  InputPortWidth=3  IndexOptions=Index vector (dialog)  Indices=[2]  OutputSizes=1
  Selector2 : Selector  InputPortWidth=3  IndexOptions=Index vector (dialog)  Indices=[2]  OutputSizes=1
  Sine Wave : Sin  Amplitude=waveAmp  Frequency=waveFreq  Phase=wphase  SampleTime=0
  Subsystem : Subsystem
  Sum : Sum  Inputs=++|
  Transport Delay : TransportDelay  DelayTime=5
  Conn1 : PMIOPort  Port=1  Side=Left
  toe_pos : Outport
  wires:
  Body Sensor1/2 -> Selector2/1
  Selector1/1 -> Sum/2, Scope3/1, toe_pos/1  "toe pos"
  Selector2/1 -> Subsystem/2(vel)
  Subsystem/1(force) -> Scope1/1, Mux1/2  "force"
  Mux1/1 -> Body Actuator/1
  Constant/1 -> Mux1/1, Mux1/3
  PVA/1 -> Joint Actuator/1
  Body Sensor1/1 -> Selector1/1
  Sine Wave/1 -> Transport Delay/1
  Sum/1 -> Subsystem/1(pos)
  Transport Delay/1 -> Sum/1
  connections:
  Body1/LConn1 -- Prismatic1/RConn1
  Body Actuator/RConn1 -- Body1/RConn1
  Body Sensor1/LConn1 -- Body1/RConn2
  Prismatic1/LConn1 -- Conn1/RConn1
  Joint Actuator/RConn1 -- Prismatic1/LConn2

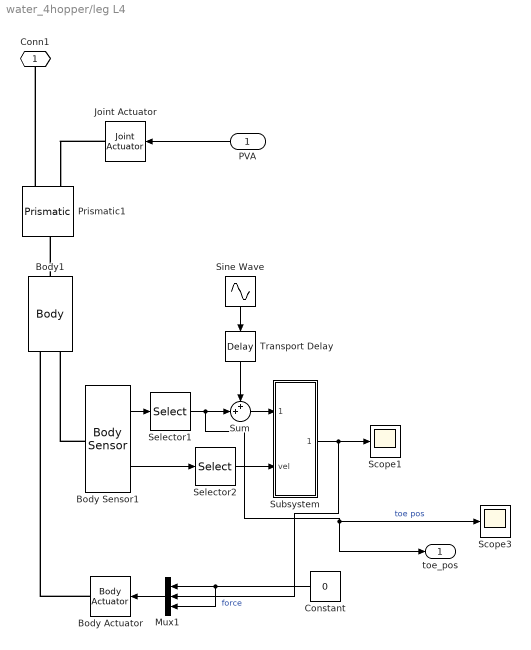
== system water_4hopper/leg L4 ==
  PVA : Inport
  Body Actuator : mblibv1/Sensors &  Actuators/Body Actuator  UpdateFromCAD=off  PhysicalDomain=Mechanical  PortType=blob  ActuationStyle=Force  AngleUnits=deg  ArcVelocityUnits=deg/s  ArcAccelerationUnits=deg/s^2  CoordPositionUnits=m  VelocityUnits=m/s  AccelerationUnits=m/s^2  ForceUnits=N  TorqueUnits=N*m  ActiveIO=on  Width=3  DialogClass=MechanicalActuatorBlock  ReferenceFrame=Local (Body CS)  Angle=off  CoordPosition=on  Force=on  Torque=off
  Body Sensor1 : mblibv1/Sensors &  Actuators/Body Sensor  UpdateFromCAD=off  PhysicalDomain=Mechanical  PortType=blob  Muxed=off  Pose=off  Angle=on  AngleUnits=deg  ArcVelocity=off  ArcVelocityUnits=deg/s  ArcAcceleration=off  ArcAccelerationUnits=deg/s^2  CoordPosition=on  CoordPositionUnits=m  Velocity=on  VelocityUnits=m/s  Acceleration=off  AccelerationUnits=m/s^2  Quaternion=on  QuaternionDT=off  QuaternionDDT=off  QuaternionUnits=off  OutputVector=[1]  ActiveIO=on  Width=6  DialogClass=MechanicalSensorBlock  ReferenceFrame=Absolute (World)
  Body1 : mblibv1/Bodies/Body  LConnTagsString=CS1  RConnTagsString=CS2|CS3  UpdateFromCAD=off  DialogClass=MechanicalBodyBlock  Mass=0  MassUnits=kg  InertiaUnits=kg*m^2  Inertia=zeros(3)  Shape=Cylinder  ShapeDims=[1 1]  ShapeUnits=m  ShapeUse=false  Density=1  DensityUnits=kg/m^3  DensityUse=false  GraphicsMode=MACHINE_DEFAULT  BodyColorSelMode=MACHINE_DEFAULT  BodyColor=[1 0 0]  AttachedToCS=CG  CG=Left$CG$[0 -leg_length 0]$CS1$CS1$m$[0 0 0]$Euler X-Y-Z$deg$WORLD$false$none  WorkingFrames=Left$CS1$[0 0 0]$Adjoining$Adjoining$m$[0 0 0]$Euler X-Y-Z$deg$WORLD$true$none#Right$CS2$[0 -leg_length 0]$CS1$CS1$m$[0 0 0]$Euler X-Y-Z$deg$WORLD$true$none#Right$CS3$[0 -leg_length 0]$CS1$CS1$m$[0 0 0]$Euler X-Y-Z$deg$WORLD$true$none  CGPos=[0 -leg_length 0]  CGRot=[0 0 0]  CS0Pos=[]  CS0Rot=[]  CS1Pos=[0 0 0]  CS1Rot=[0 0 0]  CS2Pos=[0 -leg_length 0]  CS2Rot=[0 0 0]  CS3Pos=[0 -leg_length 0]  CS3Rot=[0 0 0]  CS4Pos=[]  CS4Rot=[]  CS5Pos=[]  CS5Rot=[]  CS6Pos=[]  CS6Rot=[]  CS7Pos=[]  CS7Rot=[]  CS8Pos=[]  CS8Rot=[]  CS9Pos=[]  CS9Rot=[]  CS10Pos=[]  CS10Rot=[]  CS11Pos=[]  CS11Rot=[]  CS12Pos=[]  CS12Rot=[]  CS13Pos=[]  CS13Rot=[]  CS14Pos=[]  CS14Rot=[]  CS15Pos=[]  CS15Rot=[]  CS16Pos=[]  CS16Rot=[]  CS17Pos=[]  CS17Rot=[]  CS18Pos=[]  CS18Rot=[]  CS19Pos=[]  CS19Rot=[]  CS20Pos=[]  CS20Rot=[]
  Constant : Constant  Value=0
  Joint Actuator : mblibv1/Sensors &  Actuators/Joint Actuator  UpdateFromCAD=off  PhysicalDomain=Mechanical  PortType=blob  ActuationStyle=Motion  AngleUnits=deg  ArcVelocityUnits=deg/s  ArcAccelerationUnits=deg/s^2  CoordPositionUnits=m  VelocityUnits=m/s  AccelerationUnits=m/s^2  ForceUnits=N  TorqueUnits=N*m  ActiveIO=on  Width=3  DialogClass=MechanicalActuatorBlock  Primitive=P1  ReferenceFrame=Absolute (World)
  Mux1 : Mux  Inputs=3
  Prismatic1 : mblibv1/Joints/Prismatic  LConnTagsString=__newl0|SA1  RConnTagsString=__newr0  UpdateFromCAD=off  NumSAPorts=1  CutJoint=off  MarkAsCut=off  Primitives=prismatic  PrimitiveProps=P1$World$[0 1 0]$prismatic  DialogClass=JointBlock  P1Axis=[0 1 0]
  Scope1 : Scope
      settings: SaveName=force_L
  Scope3 : Scope
      settings: SaveName=toe_position_L
  Selector1 : Selector  InputPortWidth=3  IndexOptions=Index vector (dialog)  Indices=[2]  OutputSizes=1
  Selector2 : Selector  InputPortWidth=3  IndexOptions=Index vector (dialog)  Indices=[2]  OutputSizes=1
  Sine Wave : Sin  Amplitude=waveAmp  Frequency=waveFreq  Phase=wphase  SampleTime=0
  Subsystem : Subsystem
  Sum : Sum  Inputs=++|
  Transport Delay : TransportDelay  DelayTime=5
  Conn1 : PMIOPort  Port=1  Side=Left
  toe_pos : Outport
  wires:
  Body Sensor1/2 -> Selector2/1
  Selector1/1 -> Sum/2, Scope3/1, toe_pos/1  "toe pos"
  Selector2/1 -> Subsystem/2(vel)
  Subsystem/1(force) -> Scope1/1, Mux1/2  "force"
  Mux1/1 -> Body Actuator/1
  Constant/1 -> Mux1/1, Mux1/3
  PVA/1 -> Joint Actuator/1
  Body Sensor1/1 -> Selector1/1
  Sine Wave/1 -> Transport Delay/1
  Sum/1 -> Subsystem/1(pos)
  Transport Delay/1 -> Sum/1
  connections:
  Body1/LConn1 -- Prismatic1/RConn1
  Body Actuator/RConn1 -- Body1/RConn1
  Body Sensor1/LConn1 -- Body1/RConn2
  Prismatic1/LConn1 -- Conn1/RConn1
  Joint Actuator/RConn1 -- Prismatic1/LConn2

== system water_4hopper/CPG_Network2/FL_HL lag ==
  In1 : Inport
  In2 : Inport  Port=2
  Constant : Constant  Value=d_phase
  Gain : Gain  Gain=-1
  Sum : Sum  Inputs=--+
  sin : Fcn  Expr=coupling_weight*sin(u(1))
  Out1 : Outport
  Out2 : Outport  Port=2
  wires:
  Sum/1 -> sin/1
  sin/1 -> Gain/1, Out1/1
  Constant/1 -> Sum/2
  In1/1 -> Sum/1
  In2/1 -> Sum/3
  Gain/1 -> Out2/1

== system water_4hopper/CPG_Network2/FR_FL lag ==
  In1 : Inport
  In2 : Inport  Port=2
  Constant : Constant  Value=d_phase
  Gain : Gain  Gain=-1
  Sum : Sum  Inputs=--+
  sin : Fcn  Expr=coupling_weight*sin(u(1))
  Out1 : Outport
  Out2 : Outport  Port=2
  wires:
  Sum/1 -> sin/1
  sin/1 -> Gain/1, Out1/1
  Constant/1 -> Sum/2
  In1/1 -> Sum/1
  In2/1 -> Sum/3
  Gain/1 -> Out2/1

== system water_4hopper/CPG_Network2/FR_HR lag ==
  In1 : Inport
  In2 : Inport  Port=2
  Constant : Constant  Value=d_phase
  Gain : Gain  Gain=-1
  Sum : Sum  Inputs=--+
  sin : Fcn  Expr=coupling_weight*sin(u(1))
  Out1 : Outport
  Out2 : Outport  Port=2
  wires:
  Gain/1 -> Out2/1
  In2/1 -> Sum/3
  In1/1 -> Sum/1
  Constant/1 -> Sum/2
  sin/1 -> Out1/1, Gain/1
  Sum/1 -> sin/1

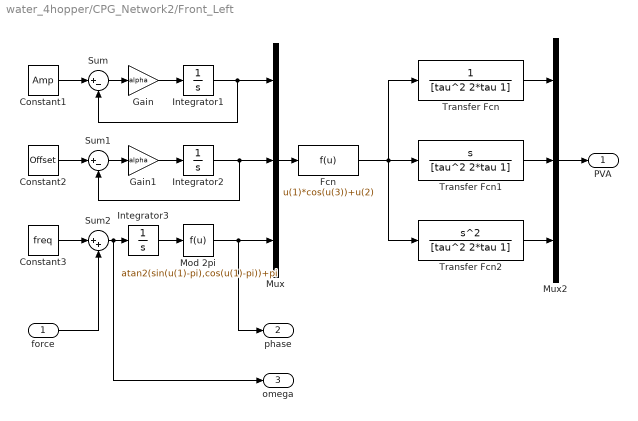
== system water_4hopper/CPG_Network2/Front_Left ==
  force : Inport
  Constant1 : Constant  Value=Amp
  Constant2 : Constant  Value=Offset
  Constant3 : Constant  Value=freq
  Fcn : Fcn  Expr=u(1)*cos(u(3))+u(2)
  Gain : Gain  Gain=alpha
  Gain1 : Gain  Gain=alpha
  Integrator1 : Integrator
  Integrator2 : Integrator
  Integrator3 : Integrator  InitialCondition=init_phi + 0.01*rand
  Mod 2pi : Fcn  Expr=atan2(sin(u(1)-pi),cos(u(1)-pi))+pi
  Mux : Mux  Inputs=3
  Mux2 : Mux  Inputs=3
  Sum : Sum  Inputs=|+-
  Sum1 : Sum  Inputs=|+-
  Sum2 : Sum  Inputs=|++
  Transfer Fcn : TransferFcn  Denominator=[tau^2 2*tau 1]
  Transfer Fcn1 : TransferFcn  Numerator=[1 0]  Denominator=[tau^2 2*tau 1]
  Transfer Fcn2 : TransferFcn  Numerator=[1 0 0]  Denominator=[tau^2 2*tau 1]
  PVA : Outport
  phase : Outport  Port=2
  omega : Outport  Port=3
  wires:
  Sum/1 -> Gain/1
  Integrator1/1 -> Sum/2, Mux/1
  Constant1/1 -> Sum/1
  Gain/1 -> Integrator1/1
  Sum1/1 -> Gain1/1
  Integrator2/1 -> Sum1/2, Mux/2
  Constant2/1 -> Sum1/1
  Gain1/1 -> Integrator2/1
  Mux/1 -> Fcn/1
  Mod 2pi/1 -> phase/1, Mux/3
  Integrator3/1 -> Mod 2pi/1
  Constant3/1 -> Sum2/1
  Sum2/1 -> omega/1, Integrator3/1
  force/1 -> Sum2/2
  Transfer Fcn2/1 -> Mux2/3
  Transfer Fcn/1 -> Mux2/1
  Transfer Fcn1/1 -> Mux2/2
  Fcn/1 -> Transfer Fcn2/1, Transfer Fcn/1, Transfer Fcn1/1
  Mux2/1 -> PVA/1

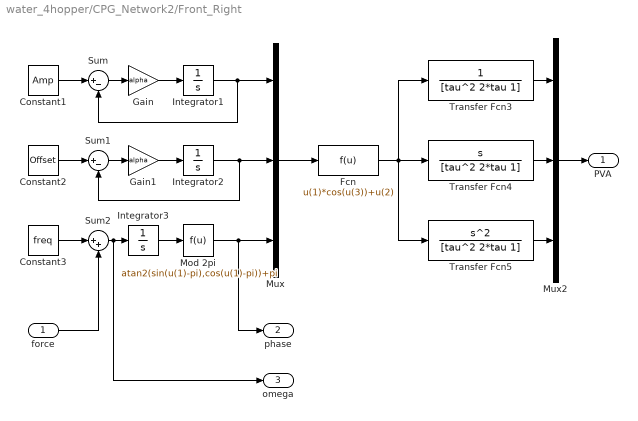
== system water_4hopper/CPG_Network2/Front_Right ==
  force : Inport
  Constant1 : Constant  Value=Amp
  Constant2 : Constant  Value=Offset
  Constant3 : Constant  Value=freq
  Fcn : Fcn  Expr=u(1)*cos(u(3))+u(2)
  Gain : Gain  Gain=alpha
  Gain1 : Gain  Gain=alpha
  Integrator1 : Integrator
  Integrator2 : Integrator
  Integrator3 : Integrator  InitialCondition=init_phi + 0.01*rand
  Mod 2pi : Fcn  Expr=atan2(sin(u(1)-pi),cos(u(1)-pi))+pi
  Mux : Mux  Inputs=3
  Mux2 : Mux  Inputs=3
  Sum : Sum  Inputs=|+-
  Sum1 : Sum  Inputs=|+-
  Sum2 : Sum  Inputs=|++
  Transfer Fcn3 : TransferFcn  Denominator=[tau^2 2*tau 1]
  Transfer Fcn4 : TransferFcn  Numerator=[1 0]  Denominator=[tau^2 2*tau 1]
  Transfer Fcn5 : TransferFcn  Numerator=[1 0 0]  Denominator=[tau^2 2*tau 1]
  PVA : Outport
  phase : Outport  Port=2
  omega : Outport  Port=3
  wires:
  Sum/1 -> Gain/1
  Integrator1/1 -> Sum/2, Mux/1
  Constant1/1 -> Sum/1
  Gain/1 -> Integrator1/1
  Sum1/1 -> Gain1/1
  Integrator2/1 -> Sum1/2, Mux/2
  Constant2/1 -> Sum1/1
  Gain1/1 -> Integrator2/1
  Mux/1 -> Fcn/1
  Mod 2pi/1 -> phase/1, Mux/3
  Integrator3/1 -> Mod 2pi/1
  Constant3/1 -> Sum2/1
  Sum2/1 -> omega/1, Integrator3/1
  force/1 -> Sum2/2
  Mux2/1 -> PVA/1
  Fcn/1 -> Transfer Fcn5/1, Transfer Fcn3/1, Transfer Fcn4/1
  Transfer Fcn3/1 -> Mux2/1
  Transfer Fcn4/1 -> Mux2/2
  Transfer Fcn5/1 -> Mux2/3

== system water_4hopper/CPG_Network2/HR_HL lag ==
  In1 : Inport
  In2 : Inport  Port=2
  Constant : Constant  Value=d_phase
  Gain : Gain  Gain=-1
  Sum : Sum  Inputs=--+
  sin : Fcn  Expr=coupling_weight*sin(u(1))
  Out1 : Outport
  Out2 : Outport  Port=2
  wires:
  Gain/1 -> Out2/1
  In2/1 -> Sum/3
  In1/1 -> Sum/1
  Constant/1 -> Sum/2
  sin/1 -> Out1/1, Gain/1
  Sum/1 -> sin/1

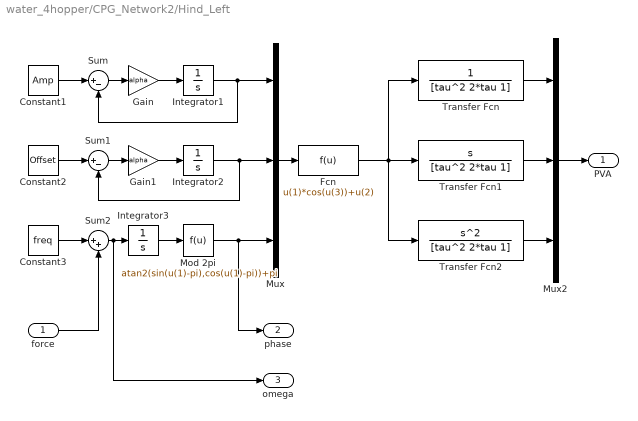
== system water_4hopper/CPG_Network2/Hind_Left ==
  force : Inport
  Constant1 : Constant  Value=Amp
  Constant2 : Constant  Value=Offset
  Constant3 : Constant  Value=freq
  Fcn : Fcn  Expr=u(1)*cos(u(3))+u(2)
  Gain : Gain  Gain=alpha
  Gain1 : Gain  Gain=alpha
  Integrator1 : Integrator
  Integrator2 : Integrator
  Integrator3 : Integrator  InitialCondition=init_phi + 0.01*rand
  Mod 2pi : Fcn  Expr=atan2(sin(u(1)-pi),cos(u(1)-pi))+pi
  Mux : Mux  Inputs=3
  Mux2 : Mux  Inputs=3
  Sum : Sum  Inputs=|+-
  Sum1 : Sum  Inputs=|+-
  Sum2 : Sum  Inputs=|++
  Transfer Fcn : TransferFcn  Denominator=[tau^2 2*tau 1]
  Transfer Fcn1 : TransferFcn  Numerator=[1 0]  Denominator=[tau^2 2*tau 1]
  Transfer Fcn2 : TransferFcn  Numerator=[1 0 0]  Denominator=[tau^2 2*tau 1]
  PVA : Outport
  phase : Outport  Port=2
  omega : Outport  Port=3
  wires:
  Sum/1 -> Gain/1
  Integrator1/1 -> Sum/2, Mux/1
  Constant1/1 -> Sum/1
  Gain/1 -> Integrator1/1
  Sum1/1 -> Gain1/1
  Integrator2/1 -> Sum1/2, Mux/2
  Constant2/1 -> Sum1/1
  Gain1/1 -> Integrator2/1
  Mux/1 -> Fcn/1
  Mod 2pi/1 -> phase/1, Mux/3
  Integrator3/1 -> Mod 2pi/1
  Constant3/1 -> Sum2/1
  Sum2/1 -> omega/1, Integrator3/1
  force/1 -> Sum2/2
  Transfer Fcn2/1 -> Mux2/3
  Transfer Fcn/1 -> Mux2/1
  Transfer Fcn1/1 -> Mux2/2
  Fcn/1 -> Transfer Fcn2/1, Transfer Fcn/1, Transfer Fcn1/1
  Mux2/1 -> PVA/1

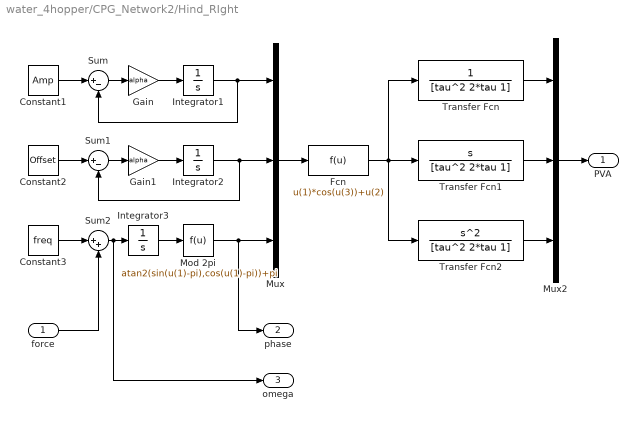
== system water_4hopper/CPG_Network2/Hind_RIght ==
  force : Inport
  Constant1 : Constant  Value=Amp
  Constant2 : Constant  Value=Offset
  Constant3 : Constant  Value=freq
  Fcn : Fcn  Expr=u(1)*cos(u(3))+u(2)
  Gain : Gain  Gain=alpha
  Gain1 : Gain  Gain=alpha
  Integrator1 : Integrator
  Integrator2 : Integrator
  Integrator3 : Integrator  InitialCondition=init_phi + 0.01*rand
  Mod 2pi : Fcn  Expr=atan2(sin(u(1)-pi),cos(u(1)-pi))+pi
  Mux : Mux  Inputs=3
  Mux2 : Mux  Inputs=3
  Sum : Sum  Inputs=|+-
  Sum1 : Sum  Inputs=|+-
  Sum2 : Sum  Inputs=|++
  Transfer Fcn : TransferFcn  Denominator=[tau^2 2*tau 1]
  Transfer Fcn1 : TransferFcn  Numerator=[1 0]  Denominator=[tau^2 2*tau 1]
  Transfer Fcn2 : TransferFcn  Numerator=[1 0 0]  Denominator=[tau^2 2*tau 1]
  PVA : Outport
  phase : Outport  Port=2
  omega : Outport  Port=3
  wires:
  Sum/1 -> Gain/1
  Integrator1/1 -> Sum/2, Mux/1
  Constant1/1 -> Sum/1
  Gain/1 -> Integrator1/1
  Sum1/1 -> Gain1/1
  Integrator2/1 -> Sum1/2, Mux/2
  Constant2/1 -> Sum1/1
  Gain1/1 -> Integrator2/1
  Mux/1 -> Fcn/1
  Mod 2pi/1 -> phase/1, Mux/3
  Integrator3/1 -> Mod 2pi/1
  Constant3/1 -> Sum2/1
  Sum2/1 -> omega/1, Integrator3/1
  force/1 -> Sum2/2
  Transfer Fcn2/1 -> Mux2/3
  Transfer Fcn/1 -> Mux2/1
  Transfer Fcn1/1 -> Mux2/2
  Fcn/1 -> Transfer Fcn2/1, Transfer Fcn/1, Transfer Fcn1/1
  Mux2/1 -> PVA/1

== system water_4hopper/CPG_Network2/split FL ==
  w_pos : Inport
  PVA : Inport  Port=2
  w_neg : Inport  Port=3
  Product : Product  RndMeth=Zero
  Product1 : Product  RndMeth=Zero
  Sum2 : Sum  Inputs=|++
  enable : Subsystem
  sel : Selector  InputPortWidth=3  IndexOptions=Index vector (dialog)  Indices=[2]  OutputSizes=1
  Force : Outport
  wires:
  Product/1 -> Sum2/1
  w_pos/1 -> Product/1
  w_neg/1 -> Product1/1
  Product1/1 -> Sum2/2
  PVA/1 -> sel/1
  enable/1(pos) -> Product/2
  enable/2(neg) -> Product1/2
  Sum2/1 -> Force/1
  sel/1 -> enable/1(in)

== system water_4hopper/CPG_Network2/split FL1 ==
  w_pos : Inport
  PVA : Inport  Port=2
  w_neg : Inport  Port=3
  Product : Product  RndMeth=Zero
  Product1 : Product  RndMeth=Zero
  Sum2 : Sum  Inputs=|++
  enable : Subsystem
  sel : Selector  InputPortWidth=3  IndexOptions=Index vector (dialog)  Indices=[2]  OutputSizes=1
  Force : Outport
  wires:
  sel/1 -> enable/1(in)
  Sum2/1 -> Force/1
  enable/2(neg) -> Product1/2
  enable/1(pos) -> Product/2
  PVA/1 -> sel/1
  Product1/1 -> Sum2/2
  w_neg/1 -> Product1/1
  w_pos/1 -> Product/1
  Product/1 -> Sum2/1

== system water_4hopper/CPG_Network2/split FL2 ==
  w_pos : Inport
  PVA : Inport  Port=2
  w_neg : Inport  Port=3
  Product : Product  RndMeth=Zero
  Product1 : Product  RndMeth=Zero
  Sum2 : Sum  Inputs=|++
  enable : Subsystem
  sel : Selector  InputPortWidth=3  IndexOptions=Index vector (dialog)  Indices=[2]  OutputSizes=1
  Force : Outport
  wires:
  Product/1 -> Sum2/1
  w_pos/1 -> Product/1
  w_neg/1 -> Product1/1
  Product1/1 -> Sum2/2
  PVA/1 -> sel/1
  enable/1(pos) -> Product/2
  enable/2(neg) -> Product1/2
  Sum2/1 -> Force/1
  sel/1 -> enable/1(in)

== system water_4hopper/CPG_Network2/split FL3 ==
  w_pos : Inport
  PVA : Inport  Port=2
  w_neg : Inport  Port=3
  Product : Product  RndMeth=Zero
  Product1 : Product  RndMeth=Zero
  Sum2 : Sum  Inputs=|++
  enable : Subsystem
  sel : Selector  InputPortWidth=3  IndexOptions=Index vector (dialog)  Indices=[2]  OutputSizes=1
  Force : Outport
  wires:
  Product/1 -> Sum2/1
  w_pos/1 -> Product/1
  w_neg/1 -> Product1/1
  Product1/1 -> Sum2/2
  PVA/1 -> sel/1
  enable/1(pos) -> Product/2
  enable/2(neg) -> Product1/2
  Sum2/1 -> Force/1
  sel/1 -> enable/1(in)

== system water_4hopper/Controller/PID ==
  output_err : Inport
  Derivative Gain : Gain  Gain=D  Multiplication=Matrix(K*u)
  Gain : Gain  Gain=Filter_Coef
  Integral Gain : Gain  DisableCoverage=on  Gain=I  Multiplication=Matrix(K*u)
  Integrator : Integrator
  Integrator1 : Integrator
  Proportional Gain : Gain  Gain=P  Multiplication=Matrix(K*u)
  Sum : Sum  Inputs=|+-
  Sum11 : Sum  Inputs=+++
  accel_des : Outport
  wires:
  Proportional Gain/1 -> Sum11/1
  Sum11/1 -> accel_des/1
  Integrator/1 -> Sum11/2
  Gain/1 -> Integrator1/1, Sum11/3
  output_err/1 -> Derivative Gain/1, Integral Gain/1, Proportional Gain/1
  Derivative Gain/1 -> Sum/1
  Sum/1 -> Gain/1
  Integrator1/1 -> Sum/2
  Integral Gain/1 -> Integrator/1

== system water_4hopper/Controller/Prefer Duty Factor ==
  omega : Inport
  Demux1 : Demux  Outputs=8
  Mean4 : dspstat3/Mean  run=off  reset_popup=None  InputProcessing=Columns as channels (frame based)  directionMode=Each column  dimension=1  treatSBRowAsCol=on  roiEnable=off  roiType=Rectangles  roiPortion=Entire ROI  roiOutput=Individual statistics for each ROI  roiFlag=off  outputDataTypeStr=Inherit: Same as accumulator  outputLastDataTypeStr=Inherit: Same as accumulator  outputMin=[]  outputMax=[]  roundingMode=Floor  overflowMode=off
  Mean5 : dspstat3/Mean  run=off  reset_popup=None  InputProcessing=Columns as channels (frame based)  directionMode=Each column  dimension=1  treatSBRowAsCol=on  roiEnable=off  roiType=Rectangles  roiPortion=Entire ROI  roiOutput=Individual statistics for each ROI  roiFlag=off  outputDataTypeStr=Inherit: Same as accumulator  outputLastDataTypeStr=Inherit: Same as accumulator  outputMin=[]  outputMax=[]  roundingMode=Floor  overflowMode=off
  Mux1 : Mux  Inputs=8
  Mux6 : Mux
  Mux7 : Mux
  omega _0 : Outport
  wires:
  Mean4/1 -> Mux1/3, Mux1/4, Mux1/1, Mux1/2
  Demux1/6 -> Mux7/2
  Demux1/3 -> Mux6/3
  Demux1/5 -> Mux7/1
  Mux1/1 -> omega _0/1
  Demux1/8 -> Mux7/4
  Demux1/1 -> Mux6/1
  Demux1/7 -> Mux7/3
  Demux1/4 -> Mux6/4
  omega/1 -> Demux1/1
  Mean5/1 -> Mux1/7, Mux1/8, Mux1/5, Mux1/6
  Mux7/1 -> Mean5/1
  Mux6/1 -> Mean4/1
  Demux1/2 -> Mux6/2

== system water_4hopper/Controller/Prefer No Duty Factor ==
  omega : Inport
  Demux1 : Demux  Outputs=8
  Mean{1..3,8} (4 alike) : dspstat3/Mean  run=off  reset_popup=None  InputProcessing=Columns as channels (frame based)  directionMode=Each column  dimension=1  treatSBRowAsCol=on  roiEnable=off  roiType=Rectangles  roiPortion=Entire ROI  roiOutput=Individual statistics for each ROI  roiFlag=off  outputDataTypeStr=Inherit: Same as accumulator  outputLastDataTypeStr=Inherit: Same as accumulator  outputMin=[]  outputMax=[]  roundingMode=Floor  overflowMode=off
  Mux1 : Mux  Inputs=8
  Mux{2..5} (4 alike) : Mux  Inputs=2
  omega_0 : Outport
  wires:
  Demux1/7 -> Mux4/2
  Demux1/1 -> Mux2/1
  Demux1/6 -> Mux3/2
  Mux2/1 -> Mean1/1
  Mux4/1 -> Mean3/1
  Mux3/1 -> Mean2/1
  Demux1/2 -> Mux3/1
  Mean3/1 -> Mux1/7, Mux1/3
  Demux1/5 -> Mux2/2
  Mux1/1 -> omega_0/1
  Mean1/1 -> Mux1/5, Mux1/1
  omega/1 -> Demux1/1
  Mean2/1 -> Mux1/6, Mux1/2
  Demux1/3 -> Mux4/1
  Demux1/4 -> Mux5/1
  Mean8/1 -> Mux1/8, Mux1/4
  Demux1/8 -> Mux5/2
  Mux5/1 -> Mean8/1
